simulink model "SmartACCFilter"  (R2019b)
settings: Solver=FixedStepAuto  StartTime=0.0  StopTime=data.timeVectorAcc(end)  FixedStep=0.01  RelTol=1e-3
values from neighbouring files (symbols this model uses):
  data = logFile.getSimulationData    [convertFiles2mat.m]    (also in startupThorsten.m)
undefined symbols (not defined in the file or in its folder): timeVector
settings Model: Creator=snj7rt  LastModifiedBy=sot2fr
settings DataIOCC: ReturnWorkspaceOutputs=off
settings DebuggingCC: ArithmeticOperatorsInVariantConditions=warning
settings SFSimCC: SimUseLocalCustomCode=off  CustomCodeUndefinedFunction=UseInterfaceOnly
settings RTWCC: RTWUseLocalCustomCode=off
settings CodeAppCC: StateflowObjectComments=on

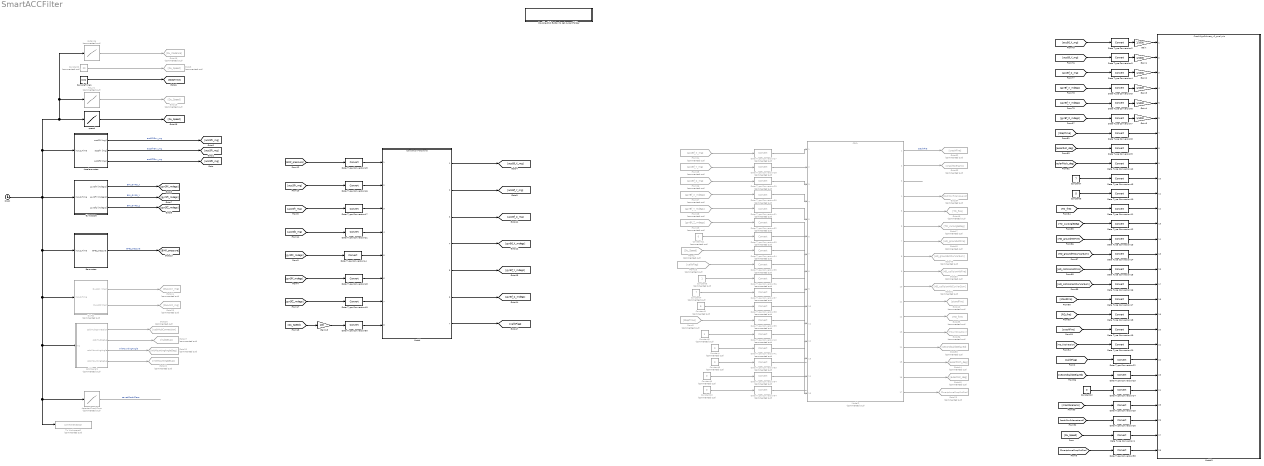
== system SmartACCFilter ==
  Acc_X1 : Lookup_n-D  Commented=on  NumberOfTableDimensions=1  BreakpointsForDimension1=timeVector(1:length([ones(floor(0.3*length(timeVector)),1);zeros(floor(0.7*length(timeVector)),1)]))  BreakpointsForDimension3=[5, 7]  Table=[20*ones(floor(0.3*length(timeVector)),1);zeros(floor(0.7*length(timeVector)),1)]  InternalRulePriority=Speed  RndMeth=Simplest  InputSameDT=on
  Accelerometer : Subsystem
  Barometer : Subsystem
  Clock : Clock
  Constant{,8..11} (5 alike) : Constant  Commented=on  Value=0
  Constant1 : Constant  Commented=on  Value=5
  Constant12 : Constant  Value=0
  Constant2 : Constant  Commented=on  Value=20
  Constant3 : Constant  Commented=on
  Constant4 : Constant  Commented=on  Value=7
  Constant5 : Constant  Commented=on
  Constant6 : Constant  Value=5
  Constant7 : Constant  Value=7
  Data Type Conversion{1..20,22..26,42..43,58} (28 alike) : DataTypeConversion
  Data Type Conversion{21,44..50} (8 alike) : DataTypeConversion  RndMeth=Zero
  Data Type Conversion{27..41,53..54,64} (18 alike) : DataTypeConversion  Commented=on  RndMeth=Zero
  Double-Click Button to set current folder : Subsystem
      settings: OpenFcn=cd(fileparts(get_param(gcs,'filename')));
      mask Display: disp('\bf\fontsize{16}Double-Click to set current folder      ','texmode','on')
  DuAcc : Subsystem  Commented=on
  From1 : From  Commented=on  GotoTag=Du_Speed
  From16 : From  Commented=on  GotoTag=calibFlag
  From24 : From  Commented=on  GotoTag=accBf_X_mg
  From25 : From  Commented=on  GotoTag=accBf_Y_mg
  From26 : From  Commented=on  GotoTag=accBf_Z_mg
  From27 : From  Commented=on  GotoTag=gyrBf_X_mdegs
  From28 : From  Commented=on  GotoTag=gyrBf_Y_mdegs
  From29 : From  Commented=on  GotoTag=gyrBf_Z_mdegs
  From5 : From  Commented=on  GotoTag=StepTime
  Gain{,1..5} (6 alike) : Gain  Gain=1/1000
  Gain13 : Gain  Gain=100
  Goto10 : Goto  Commented=on  GotoTag=standFire
  Goto16 : Goto  Commented=on  GotoTag=Du_Cadence
  Goto19 : Goto  Commented=on  GotoTag=Du_Speed
  Goto20 : Goto  Commented=on  GotoTag=initMountingAngleDeg
  Goto22 : Goto  Commented=on  GotoTag=initMountingSetup
  Goto23 : Goto  Commented=on  GotoTag=SmartphoneDropOutFire
  Goto24 : Goto  Commented=on  GotoTag=DuAccX_mg
  Goto25 : Goto  Commented=on  GotoTag=DuAccZ_mg
  Goto26 : Goto  Commented=on  GotoTag=cobiHubConnection
  Goto27 : Goto  Commented=on  GotoTag=hubSetup
  Goto3 : Goto  Commented=on  GotoTag=Du_Speed
  Goto44 : Goto  Commented=on  GotoTag=eulerPitch_deg
  Goto45 : Goto  Commented=on  GotoTag=eulerRoll_deg
  Goto46 : Goto  Commented=on  GotoTag=TO_fire
  Goto47 : Goto  Commented=on  GotoTag=TO_curAngleDeg
  Goto48 : Goto  Commented=on  GotoTag=HD_groundHitFire
  Goto49 : Goto  Commented=on  GotoTag=HD_groundHitCurVarSum
  Goto50 : Goto  Commented=on  GotoTag=HD_collisionHitFire
  Goto51 : Goto  Commented=on  GotoTag=HD_collisionHitCurVarSum
  Goto52 : Goto  Commented=on  GotoTag=crashFire
  Goto53 : Goto  Commented=on  GotoTag=crashScenario
  Goto54 : Goto  Commented=on  GotoTag=crashConfidenceLevel
  Goto55 : Goto  Commented=on  GotoTag=RD_fire
  Goto56 : Goto  Commented=on  GotoTag=HD_hitDirection
  Goto58 : Goto  Commented=on  GotoTag=secondCalibDelayed
  Gyroscope : Subsystem
  Model : ModelReference  ModelNameDialog=CalibrationMotorbike.slx  SimulationMode=Normal  ModelReferenceVersion=1.1435
  Model2 : ModelReference  Commented=on  ModelNameDialog=CRCL.slx  SimulationMode=Normal  ModelReferenceVersion=1.1927
  Model3 : ModelReference  ModelNameDialog=CrashAlgoSchnee_v2_analysis.slx  SimulationMode=Normal  ModelReferenceVersion=1.56
  SampleTime1 : Constant  Value=0.01
  To Workspace2 : ToWorkspace  Commented=on  VariableName=simTimeVector  SampleTime=-1
      settings: Save2DSignal=2-D array (concatenate along first dimension)
  cadence : Lookup_n-D  Commented=on  NumberOfTableDimensions=1  BreakpointsForDimension1=data.timeVectorAcc  BreakpointsForDimension3=[5, 7]  Table=data.cadence_rpm  InternalRulePriority=Speed  RndMeth=Simplest  InputSameDT=on
  cobiSignals : Subsystem  Commented=on
  detectedCrashClass : Lookup_n-D  Commented=on  NumberOfTableDimensions=1  BreakpointsForDimension1=data.timeVectorAcc  BreakpointsForDimension3=[5, 7]  Table=data.crashClass  InternalRulePriority=Speed  RndMeth=Simplest  InputSameDT=on
  speed : Lookup_n-D  NumberOfTableDimensions=1  BreakpointsForDimension1=data.timeVectorAcc  BreakpointsForDimension3=[5, 7]  Table=data.speed_kmh  InternalRulePriority=Speed  RndMeth=Simplest  InputSameDT=on
  wires:
  Accelerometer/1(accSfX [mg]) -> [accSfX_mg]  "accSfXEnv_mg"
  Accelerometer/2(accSfY [mg]) -> [accSfY_mg]  "accSfYEnv_mg"
  Accelerometer/3(accSfZ [mg]) -> [accSfZ_mg]  "accSfZEnv_mg"
  Clock/1 -> cadence/1, Acc_X1/1, speed/1, Accelerometer/1(input_Time), Gyroscope/1(input_Time), DuAcc/1(input_Time), To Workspace2/1, detectedCrashClass/1, cobiSignals/1(In1), Barometer/1(input_Time)
  SampleTime1/1 -> [StepTime]
  Gyroscope/2(gyrSfY [mdeg/s]) -> [gyrSfY_mdegs]  "BMI_GYRO_Y"
  Gyroscope/1(gyrSfX [mdeg/s]) -> [gyrSfX_mdegs]  "BMI_GYRO_X"
  Gyroscope/3(gyrSfZ [mdeg/s]) -> [gyrSfZ_mdegs]  "BMI_GYRO_Z"
  Barometer/1(BME_pressure) -> [BMP_pressure]  "BME_pressure"
  Data Type Conversion14/1 -> Model3/15
  Constant4/1 -> Data Type Conversion37/1
  Data Type Conversion3/1 -> Gain1/1
  Data Type Conversion38/1 -> Model2/12
  Data Type Conversion16/1 -> Model3/17
  Data Type Conversion9/1 -> Model3/8
  [eulerPitch_deg] -> Data Type Conversion42/1
  Data Type Conversion31/1 -> Model2/5
  [standFire] -> Data Type Conversion17/1
  Model2/15 -> Goto44/1
  Constant12/1 -> Data Type Conversion24/1
  [gyrBf_Y_mdegs] -> Data Type Conversion6/1
  Data Type Conversion19/1 -> Model3/20
  From5/1 -> Data Type Conversion39/1
  Data Type Conversion36/1 -> Model2/10
  Constant1/1 -> Data Type Conversion38/1
  Data Type Conversion29/1 -> Model2/3
  Data Type Conversion8/1 -> Model3/7
  Model2/6 -> Goto47/1
  Data Type Conversion5/1 -> Gain3/1
  Data Type Conversion42/1 -> Model3/9
  [gyrBf_X_mdegs] -> Data Type Conversion5/1
  [secondCalibDelayed] -> Data Type Conversion23/1
  [gyrBf_Z_mdegs] -> Data Type Conversion7/1
  Model2/11 -> Goto10/1
  [HD_collisionHitFire] -> Data Type Conversion15/1
  Constant5/1 -> Data Type Conversion36/1
  Model2/9 -> Goto50/1
  Data Type Conversion11/1 -> Model3/12
  Model2/8 -> Goto49/1
  Data Type Conversion28/1 -> Model2/2
  Model2/13 -> Goto56/1
  [calibFlag] -> Data Type Conversion22/1
  Data Type Conversion7/1 -> Gain5/1
  [HD_groundHitFire] -> Data Type Conversion13/1
  [HD_groundHitCurVarSum] -> Data Type Conversion14/1
  Model2/10 -> Goto51/1
  Model2/5 -> Goto46/1
  Data Type Conversion37/1 -> Model2/11
  [crashConfidenceLevel] -> Data Type Conversion26/1
  From1/1 -> Data Type Conversion34/1
  [crashFire] -> Data Type Conversion19/1
  [StepTime] -> Data Type Conversion8/1
  Data Type Conversion32/1 -> Model2/6
  Model2/7 -> Goto48/1
  Constant7/1 -> Data Type Conversion43/1
  Model2/16 -> Goto45/1
  Data Type Conversion43/1 -> Model3/10
  Data Type Conversion20/1 -> Model3/21
  Data Type Conversion15/1 -> Model3/16
  Constant6/1 -> Data Type Conversion10/1
  Data Type Conversion34/1 -> Model2/8
  Data Type Conversion27/1 -> Model2/1
  Data Type Conversion22/1 -> Model3/22
  Data Type Conversion23/1 -> Model3/23
  [RD_fire] -> Data Type Conversion18/1
  Model2/14 -> Goto58/1
  Data Type Conversion39/1 -> Model2/13
  Data Type Conversion30/1 -> Model2/4
  Constant11/1 -> Data Type Conversion33/1
  Data Type Conversion17/1 -> Model3/18
  Data Type Conversion10/1 -> Model3/11
  Data Type Conversion6/1 -> Gain4/1
  [TO_curAngleDeg] -> Data Type Conversion12/1
  Data Type Conversion24/1 -> Model3/24
  Data Type Conversion25/1 -> Model3/25
  [HD_collisionHitCurVarSum] -> Data Type Conversion16/1
  [TO_fire] -> Data Type Conversion11/1
  [accBf_Z_mg] -> Data Type Conversion4/1
  Model2/12 -> Goto55/1
  Data Type Conversion2/1 -> Gain/1
  Data Type Conversion18/1 -> Model3/19
  [accBf_X_mg] -> Data Type Conversion2/1
  Model2/4 -> Goto54/1
  Model2/1 -> Goto52/1  "CrashFire"
  Data Type Conversion13/1 -> Model3/14
  Data Type Conversion35/1 -> Model2/9
  [eulerRoll_deg] -> Data Type Conversion9/1
  Data Type Conversion4/1 -> Gain2/1
  [accBf_Y_mg] -> Data Type Conversion3/1
  Data Type Conversion26/1 -> Model3/26
  From16/1 -> Data Type Conversion35/1
  [HD_hitDirection] -> Data Type Conversion20/1
  Data Type Conversion33/1 -> Model2/7
  Data Type Conversion12/1 -> Model3/13
  [Du_Speed] -> Data Type Conversion1/1
  Data Type Conversion1/1 -> Model3/27
  [BMP_pressure] -> Data Type Conversion45/1
  Data Type Conversion45/1 -> Model/1
  Data Type Conversion46/1 -> Model/2
  Data Type Conversion47/1 -> Model/3
  Data Type Conversion21/1 -> Model/4
  Data Type Conversion44/1 -> Model/5
  Data Type Conversion48/1 -> Model/6
  Data Type Conversion49/1 -> Model/7
  [Du_Speed] -> Gain13/1
  Data Type Conversion50/1 -> Model/8
  [gyrSfX_mdegs] -> Data Type Conversion44/1
  [gyrSfY_mdegs] -> Data Type Conversion48/1
  [gyrSfZ_mdegs] -> Data Type Conversion49/1
  Constant2/1 -> Goto3/1
  Model/1 -> [accBf_X_mg]
  Model/2 -> [accBf_Y_mg]
  Model/3 -> [accBf_Z_mg]
  Model/4 -> [gyrBf_X_mdegs]
  Model/5 -> [gyrBf_Y_mdegs]
  Model/6 -> [gyrBf_Z_mdegs]
  Model/7 -> [calibFlag]
  speed/1 -> [Du_Speed]
  Gain13/1 -> Data Type Conversion50/1
  Acc_X1/1 -> Goto19/1
  Data Type Conversion40/1 -> Model2/14
  Constant3/1 -> Data Type Conversion40/1
  Data Type Conversion41/1 -> Model2/15
  Constant/1 -> Data Type Conversion41/1
  From24/1 -> Data Type Conversion27/1
  From25/1 -> Data Type Conversion28/1
  From26/1 -> Data Type Conversion29/1
  From27/1 -> Data Type Conversion30/1
  From28/1 -> Data Type Conversion31/1
  From29/1 -> Data Type Conversion32/1
  [accSfY_mg] -> Data Type Conversion47/1
  [accSfX_mg] -> Data Type Conversion46/1
  [accSfZ_mg] -> Data Type Conversion21/1
  [SmartphoneDropOutFire] -> Data Type Conversion58/1
  Data Type Conversion58/1 -> Model3/28
  Model2/2 -> Goto53/1
  [crashScenario] -> Data Type Conversion25/1
  detectedCrashClass/1 -> ?  "savedCrashClass"
  cobiSignals/1(cobiHubConnection) -> Goto26/1
  cobiSignals/2(cobiHubSetup) -> Goto27/1
  cobiSignals/3(cobiMountingAngle) -> Goto20/1  "InitMountingAngle"
  cobiSignals/4(cobiMountingSetup) -> Goto22/1
  Constant8/1 -> Data Type Conversion53/1
  Data Type Conversion53/1 -> ?
  DuAcc/1(DuAccX  [mg]) -> Goto24/1
  DuAcc/2(DuAccZ [mg]) -> Goto25/1
  Model2/3 -> ?
  Constant10/1 -> Data Type Conversion64/1
  Data Type Conversion64/1 -> ?
  Data Type Conversion54/1 -> ?
  Constant9/1 -> Data Type Conversion54/1
  Model2/17 -> Goto23/1
  cadence/1 -> Goto16/1
  Gain/1 -> Model3/1
  Gain1/1 -> Model3/2
  Gain2/1 -> Model3/3
  Gain3/1 -> Model3/4
  Gain4/1 -> Model3/5
  Gain5/1 -> Model3/6

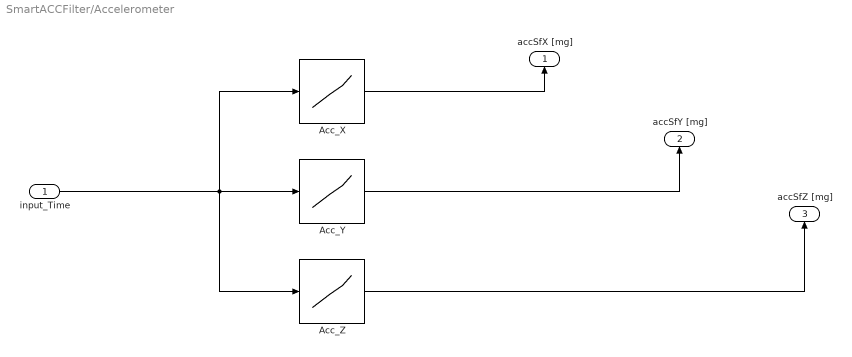
== system SmartACCFilter/Accelerometer ==
  input_Time : Inport
  Acc_X : Lookup_n-D  NumberOfTableDimensions=1  BreakpointsForDimension1=data.timeVectorAcc  BreakpointsForDimension3=[5, 7]  Table=data.AccSfX_mg  InternalRulePriority=Speed  RndMeth=Simplest  InputSameDT=on
  Acc_Y : Lookup_n-D  NumberOfTableDimensions=1  BreakpointsForDimension1=data.timeVectorAcc  BreakpointsForDimension3=[5, 7]  Table=data.AccSfY_mg  InternalRulePriority=Speed  RndMeth=Simplest  InputSameDT=on
  Acc_Z : Lookup_n-D  NumberOfTableDimensions=1  BreakpointsForDimension1=data.timeVectorAcc  BreakpointsForDimension3=[5, 7]  Table=data.AccSfZ_mg  InternalRulePriority=Speed  RndMeth=Simplest  InputSameDT=on
  accSfX [mg] : Outport  VectorParamsAs1DForOutWhenUnconnected=off
  accSfY [mg] : Outport  Port=2  VectorParamsAs1DForOutWhenUnconnected=off
  accSfZ [mg] : Outport  Port=3  VectorParamsAs1DForOutWhenUnconnected=off
  wires:
  input_Time/1 -> Acc_Z/1, Acc_Y/1, Acc_X/1
  Acc_X/1 -> accSfX [mg]/1
  Acc_Z/1 -> accSfZ [mg]/1
  Acc_Y/1 -> accSfY [mg]/1

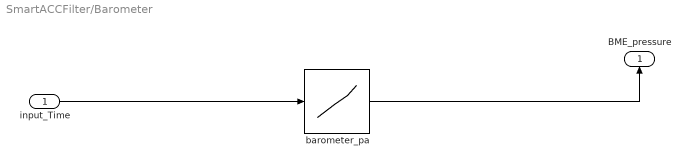
== system SmartACCFilter/Barometer ==
  input_Time : Inport
  barometer_pa : Lookup_n-D  NumberOfTableDimensions=1  BreakpointsForDimension1=data.timeVectorAcc  BreakpointsForDimension3=[5, 7]  Table=data.barometer_pa  InternalRulePriority=Speed  RndMeth=Simplest  InputSameDT=on
  BME_pressure : Outport  VectorParamsAs1DForOutWhenUnconnected=off
  wires:
  input_Time/1 -> barometer_pa/1
  barometer_pa/1 -> BME_pressure/1

== system SmartACCFilter/Double-Click Button to set current folder ==

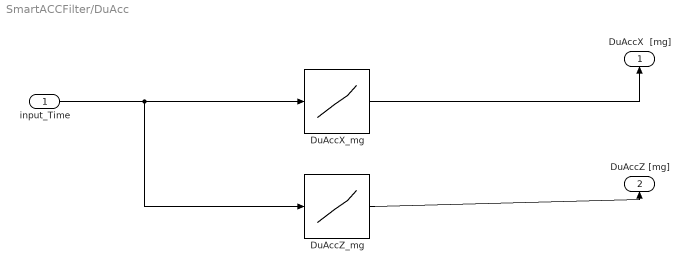
== system SmartACCFilter/DuAcc ==
  input_Time : Inport
  DuAccX_mg : Lookup_n-D  NumberOfTableDimensions=1  BreakpointsForDimension1=data.timeVectorAcc  BreakpointsForDimension3=[5, 7]  Table=data.DuAccX_mg  InternalRulePriority=Speed  RndMeth=Simplest  InputSameDT=on
  DuAccZ_mg : Lookup_n-D  NumberOfTableDimensions=1  BreakpointsForDimension1=data.timeVectorAcc  BreakpointsForDimension3=[5, 7]  Table=data.DuAccZ_mg  InternalRulePriority=Speed  RndMeth=Simplest  InputSameDT=on
  DuAccX  [mg] : Outport  VectorParamsAs1DForOutWhenUnconnected=off
  DuAccZ [mg] : Outport  Port=2  VectorParamsAs1DForOutWhenUnconnected=off
  wires:
  DuAccX_mg/1 -> DuAccX  [mg]/1
  input_Time/1 -> DuAccZ_mg/1, DuAccX_mg/1
  DuAccZ_mg/1 -> DuAccZ [mg]/1

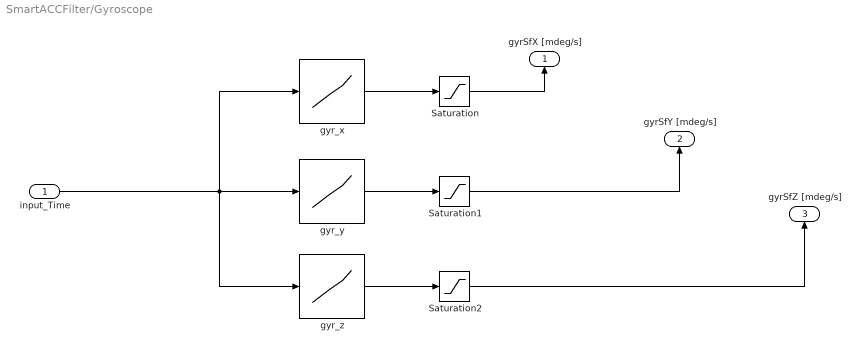
== system SmartACCFilter/Gyroscope ==
  input_Time : Inport
  Saturation : Saturate  UpperLimit=2000000  LowerLimit=-2000000
  Saturation1 : Saturate  UpperLimit=2000000  LowerLimit=-2000000
  Saturation2 : Saturate  UpperLimit=2000000  LowerLimit=-2000000
  gyr_x : Lookup_n-D  NumberOfTableDimensions=1  BreakpointsForDimension1=data.timeVectorGyr  BreakpointsForDimension3=[5, 7]  Table=data.GyrSfX_mdegs  InternalRulePriority=Speed  RndMeth=Simplest  InputSameDT=on
  gyr_y : Lookup_n-D  NumberOfTableDimensions=1  BreakpointsForDimension1=data.timeVectorGyr  BreakpointsForDimension3=[5, 7]  Table=data.GyrSfY_mdegs  InternalRulePriority=Speed  RndMeth=Simplest  InputSameDT=on
  gyr_z : Lookup_n-D  NumberOfTableDimensions=1  BreakpointsForDimension1=data.timeVectorGyr  BreakpointsForDimension3=[5, 7]  Table=data.GyrSfZ_mdegs  InternalRulePriority=Speed  RndMeth=Simplest  InputSameDT=on
  gyrSfX [mdeg/s] : Outport  VectorParamsAs1DForOutWhenUnconnected=off
  gyrSfY [mdeg/s] : Outport  Port=2  VectorParamsAs1DForOutWhenUnconnected=off
  gyrSfZ [mdeg/s] : Outport  Port=3  VectorParamsAs1DForOutWhenUnconnected=off
  wires:
  input_Time/1 -> gyr_y/1, gyr_z/1, gyr_x/1
  gyr_x/1 -> Saturation/1
  gyr_y/1 -> Saturation1/1
  gyr_z/1 -> Saturation2/1
  Saturation/1 -> gyrSfX [mdeg/s]/1
  Saturation1/1 -> gyrSfY [mdeg/s]/1
  Saturation2/1 -> gyrSfZ [mdeg/s]/1

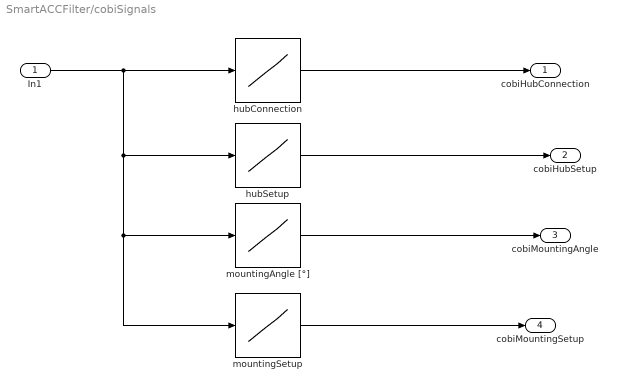
== system SmartACCFilter/cobiSignals ==
  In1 : Inport
  hubConnection : Lookup_n-D  NumberOfTableDimensions=1  BreakpointsForDimension1=data.timeVectorAcc  BreakpointsForDimension3=[5, 7]  Table=data.hubConnection  InternalRulePriority=Speed  RndMeth=Simplest  InputSameDT=on
  hubSetup : Lookup_n-D  NumberOfTableDimensions=1  BreakpointsForDimension1=data.timeVectorAcc  BreakpointsForDimension3=[5, 7]  Table=data.cobiHubSetup  InternalRulePriority=Speed  RndMeth=Simplest  InputSameDT=on
  mountingAngle [°] : Lookup_n-D  NumberOfTableDimensions=1  BreakpointsForDimension1=data.timeVectorAcc  BreakpointsForDimension3=[5, 7]  Table=data.mountingAngle  InternalRulePriority=Speed  RndMeth=Simplest  InputSameDT=on
  mountingSetup : Lookup_n-D  NumberOfTableDimensions=1  BreakpointsForDimension1=data.timeVectorAcc  BreakpointsForDimension3=[5, 7]  Table=data.mountingSetup  InternalRulePriority=Speed  RndMeth=Simplest  InputSameDT=on
  cobiHubConnection : Outport  VectorParamsAs1DForOutWhenUnconnected=off
  cobiHubSetup : Outport  Port=2  VectorParamsAs1DForOutWhenUnconnected=off
  cobiMountingAngle : Outport  Port=3  VectorParamsAs1DForOutWhenUnconnected=off
  cobiMountingSetup : Outport  Port=4  VectorParamsAs1DForOutWhenUnconnected=off
  wires:
  hubSetup/1 -> cobiHubSetup/1
  mountingSetup/1 -> cobiMountingSetup/1
  mountingAngle [°]/1 -> cobiMountingAngle/1
  In1/1 -> hubSetup/1, mountingAngle [°]/1, mountingSetup/1, hubConnection/1
  hubConnection/1 -> cobiHubConnection/1
